simulink model "sampleModel1461"  (R2023a)
settings: Solver=VariableStepAuto  StartTime=0.0  StopTime=10.0  RelTol=1e-3
libraries: hdlsllib x6
settings Model: Creator=user1  LastModifiedBy=user1

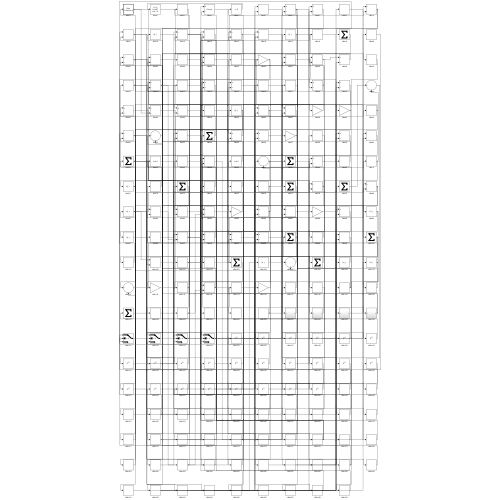
[thumbnail: Simulink's stored preview of the top-level diagram]
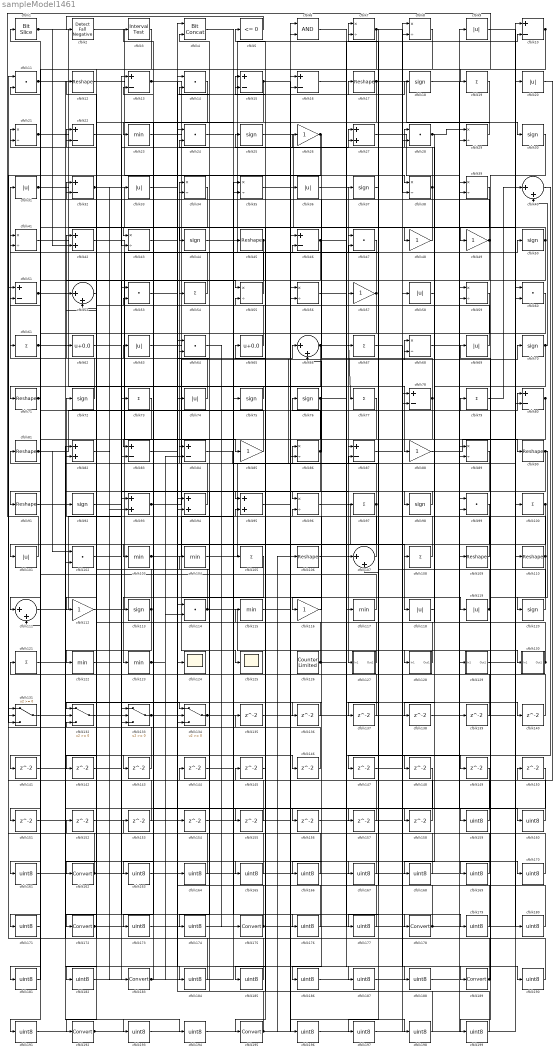
== system sampleModel1461 ==
  cfblk1 : hdlsllib/Logic and Bit Operations/Bit Slice  lidx=7  ridx=0
  cfblk{10,13,15..16,22,32,46,51,78,80,83..84,87} (13 alike) : Sum  Inputs=+-
  cfblk{19,54,61,67,73,77,79,97,100,105,108,121} (12 alike) : Sum  Inputs=+
  cfblk{9,20,31,33,36,58,63,69,74,101,118..119} (12 alike) : Abs  SaturateOnIntegerOverflow=off
  cfblk{11,14,24,28,47,53,60,64,99,102,114} (11 alike) : DotProduct  OutDataTypeStr=Inherit: Inherit via internal rule
  cfblk{23,103..104,115,117,122..123} (7 alike) : MinMax
  cfblk{12,17,45,71,81,90..91,106,109..110} (10 alike) : Reshape
  cfblk{40,52,66,107,111} (5 alike) : Sum  Inputs=|++
  cfblk{26,48..49,57,85,88,112,116} (8 alike) : Gain
  cfblk{18,25,30,37,44,50,70,72,75..76,92,98,113,120} (14 alike) : Signum
  cfblk124 : Scope
  cfblk125 : Scope
  cfblk126 : hdlsllib/Sources/Counter Limited  uplimit=7  tsamp=-1
  cfblk127 : Subsystem
      settings: LibrarySourceBlock=|
      | hdlsllib/Ports &
      | Subsystems/Subsystem
  cfblk128 : Subsystem
      settings: LibrarySourceBlock=|
      | hdlsllib/Ports &
      | Subsystems/Subsystem
  cfblk129 : Subsystem
      settings: LibrarySourceBlock=|
      | hdlsllib/Ports &
      | Subsystems/Subsystem
  cfblk130 : Subsystem
      settings: LibrarySourceBlock=|
      | hdlsllib/Ports &
      | Subsystems/Subsystem
  cfblk{131..134} (4 alike) : Switch  SaturateOnIntegerOverflow=off  InputSameDT=off
  cfblk{135..158} (24 alike) : Delay  SampleTime=1
  cfblk{159..161,163..171,173..174,176..177,179..182,184..188,190..191,193..194,196..199} (33 alike) : DataTypeConversion  OutDataTypeStr=uint8  SaturateOnIntegerOverflow=off  RndMeth=Floor
  cfblk{162,172,175,178,183,189,192,195} (8 alike) : DataTypeConversion  SaturateOnIntegerOverflow=off  RndMeth=Floor
  cfblk2 : hdlsllib/Logic and Bit Operations/Detect Fall Negative  vinit=0  OutDataTypeStr=boolean
  cfblk{7..8,21,29,34..35,38..39,41,43,55..56,59,68,86,89,96} (17 alike) : Product  Inputs=*/  RndMeth=Zero  SaturateOnIntegerOverflow=on
  cfblk{27,42,82,93..95} (6 alike) : Sum
  cfblk3 : hdlsllib/Logic and Bit Operations/Interval Test  IntervalClosedRight=on  uplimit=0.5  IntervalClosedLeft=on  lowlimit=-0.5  OutDataTypeStr=boolean
  cfblk4 : hdlsllib/Logic and Bit Operations/Bit Concat  numInputs=2
  cfblk5 : hdlsllib/Logic and Bit Operations/Compare To Zero  relop=<=  OutDataTypeStr=boolean
  cfblk6 : Logic  AllPortsSameDT=off  OutDataTypeStr=boolean
  cfblk62 : Bias  Bias=0.0  SaturateOnIntegerOverflow=off
  cfblk65 : Bias  Bias=0.0  SaturateOnIntegerOverflow=off
  wires:
  cfblk114/1 -> cfblk128/1(In1), cfblk62/1
  cfblk17/1 -> cfblk30/1, cfblk134/3
  cfblk45/1 -> cfblk151/1, cfblk163/1
  cfblk63/1 -> cfblk96/1
  cfblk120/1 -> cfblk86/1
  cfblk55/1 -> cfblk7/1
  cfblk42/1 -> cfblk85/1
  cfblk106/1 -> cfblk127/1(In1)
  cfblk84/1 -> cfblk68/1
  cfblk79/1 -> cfblk40/1
  cfblk110/1 -> cfblk72/1, cfblk169/1
  cfblk1/1 -> cfblk88/1, cfblk42/2
  cfblk23/1 -> cfblk125/1
  cfblk93/1 -> cfblk68/2, cfblk108/1
  cfblk107/1 -> cfblk5/1
  cfblk13/1 -> cfblk119/1, cfblk156/1, cfblk187/1
  cfblk50/1 -> cfblk107/1, cfblk49/1
  cfblk3/1 -> cfblk162/1
  cfblk39/1 -> cfblk195/1
  cfblk66/1 -> cfblk77/1, cfblk10/2, cfblk191/1
  cfblk14/1 -> cfblk172/1
  cfblk74/1 -> cfblk42/1
  cfblk104/1 -> cfblk20/1
  cfblk52/1 -> cfblk132/1
  cfblk12/1 -> cfblk38/1
  cfblk34/1 -> cfblk43/1
  cfblk25/1 -> cfblk48/1
  cfblk75/1 -> cfblk71/1
  cfblk113/1 -> cfblk32/2, cfblk142/1
  cfblk28/1 -> cfblk29/1, cfblk138/1
  cfblk116/1 -> cfblk96/2
  cfblk5/1 -> cfblk2/1
  cfblk65/1 -> cfblk21/1
  cfblk21/1 -> cfblk100/1, cfblk143/1
  cfblk94/1 -> cfblk12/1
  cfblk49/1 -> cfblk91/1, cfblk21/2
  cfblk38/1 -> cfblk25/1, cfblk171/1
  cfblk97/1 -> cfblk34/1, cfblk134/2
  cfblk32/1 -> cfblk124/1, cfblk93/2
  cfblk59/1 -> cfblk192/1
  cfblk130/1(Out1) -> cfblk27/1, cfblk28/1
  cfblk96/1 -> cfblk118/1
  cfblk37/1 -> cfblk107/2
  cfblk44/1 -> cfblk105/1
  cfblk72/1 -> cfblk31/1
  cfblk56/1 -> cfblk189/1
  cfblk82/1 -> cfblk183/1
  cfblk101/1 -> cfblk19/1
  cfblk133/1 -> cfblk74/1, cfblk66/1
  cfblk112/1 -> cfblk50/1
  cfblk80/1 -> cfblk182/1, cfblk185/1
  cfblk36/1 -> cfblk57/1
  cfblk51/1 -> cfblk146/1, cfblk176/1
  cfblk108/1 -> cfblk92/1
  cfblk105/1 -> cfblk123/1
  cfblk70/1 -> cfblk40/2, cfblk148/1
  cfblk86/1 -> cfblk66/2, cfblk76/1, cfblk133/3, cfblk174/1
  cfblk57/1 -> cfblk46/2, cfblk155/1
  cfblk77/1 -> cfblk87/1
  cfblk85/1 -> cfblk61/1
  cfblk22/1 -> cfblk43/2
  cfblk54/1 -> cfblk34/2
  cfblk15/1 -> cfblk103/1, cfblk157/1
  cfblk126/1 -> cfblk22/1, cfblk79/1
  cfblk91/1 -> cfblk97/1
  cfblk8/1 -> cfblk111/1
  cfblk64/1 -> cfblk175/1
  cfblk109/1 -> cfblk84/1
  cfblk41/1 -> cfblk94/2
  cfblk69/1 -> cfblk22/2
  cfblk111/1 -> cfblk33/1
  cfblk26/1 -> cfblk116/1, cfblk131/3
  cfblk123/1 -> cfblk63/1, cfblk84/2
  cfblk92/1 -> cfblk27/2
  cfblk117/1 -> cfblk41/1
  cfblk102/1 -> cfblk113/1
  cfblk78/1 -> cfblk112/1, cfblk32/1
  cfblk11/1 -> cfblk55/1, cfblk134/1
  cfblk33/1 -> cfblk15/1
  cfblk47/1 -> cfblk41/2
  cfblk88/1 -> cfblk90/1
  cfblk29/1 -> cfblk23/1
  cfblk68/1 -> cfblk29/2
  cfblk58/1 -> cfblk98/1
  cfblk98/1 -> cfblk95/1
  cfblk31/1 -> cfblk129/1(In1), cfblk188/1
  cfblk2/1 -> cfblk75/1
  cfblk119/1 -> cfblk26/1, cfblk87/2
  cfblk95/1 -> cfblk70/1
  cfblk48/1 -> cfblk44/1
  cfblk90/1 -> cfblk120/1, cfblk177/1
  cfblk43/1 -> cfblk114/1
  cfblk81/1 -> cfblk8/1, cfblk102/1, cfblk158/1
  cfblk7/1 -> cfblk38/2, cfblk47/1, cfblk52/2
  cfblk71/1 -> cfblk51/2, cfblk161/1
  cfblk100/1 -> cfblk102/2, cfblk141/1
  cfblk67/1 -> cfblk130/1(In1)
  cfblk128/1(Out1) -> cfblk95/2
  cfblk27/1 -> cfblk109/1
  cfblk103/1 -> cfblk35/2, cfblk17/1
  cfblk129/1(Out1) -> cfblk10/1
  cfblk46/1 -> cfblk133/2, cfblk140/1
  cfblk127/1(Out1) -> cfblk13/2
  cfblk60/1 -> cfblk101/1
  cfblk61/1 -> cfblk78/2, cfblk83/2, cfblk184/1
  cfblk132/1 -> cfblk80/1
  cfblk134/1 -> cfblk67/1, cfblk16/2, cfblk99/2
  cfblk19/1 -> cfblk122/1
  cfblk76/1 -> cfblk18/1, cfblk83/1
  cfblk10/1 -> cfblk28/2, cfblk137/1
  cfblk24/1 -> cfblk178/1
  cfblk135/1 -> cfblk60/2
  cfblk99/1 -> cfblk136/1
  cfblk136/1 -> cfblk132/2
  cfblk137/1 -> cfblk52/1
  cfblk138/1 -> cfblk80/2
  cfblk139/1 -> cfblk11/2
  cfblk140/1 -> cfblk15/2
  cfblk141/1 -> cfblk13/1
  cfblk142/1 -> cfblk133/1
  cfblk143/1 -> cfblk131/2
  cfblk144/1 -> cfblk35/1
  cfblk145/1 -> cfblk55/2
  cfblk146/1 -> cfblk132/3
  cfblk40/1 -> cfblk147/1
  cfblk147/1 -> cfblk78/1
  cfblk16/1 -> cfblk149/1
  cfblk20/1 -> cfblk150/1
  cfblk152/1 -> cfblk86/2
  cfblk153/1 -> cfblk131/1
  cfblk83/1 -> cfblk154/1
  cfblk154/1 -> cfblk46/1
  cfblk155/1 -> cfblk111/2
  cfblk156/1 -> cfblk8/2
  cfblk157/1 -> cfblk1/1
  cfblk158/1 -> cfblk7/2
  cfblk6/1 -> cfblk159/1
  cfblk159/1 -> cfblk65/1
  cfblk18/1 -> cfblk160/1
  cfblk160/1 -> cfblk6/1
  cfblk161/1 -> cfblk6/2
  cfblk162/1 -> cfblk152/1, cfblk9/1
  cfblk163/1 -> cfblk3/1
  cfblk53/1 -> cfblk164/1
  cfblk164/1 -> cfblk11/1
  cfblk122/1 -> cfblk165/1
  cfblk165/1 -> cfblk53/1
  cfblk148/1 -> cfblk166/1
  cfblk166/1 -> cfblk53/2
  cfblk4/1 -> cfblk167/1
  cfblk167/1 -> cfblk93/1
  cfblk118/1 -> cfblk168/1
  cfblk168/1 -> cfblk4/1
  cfblk169/1 -> cfblk4/2
  cfblk121/1 -> cfblk170/1
  cfblk170/1 -> cfblk135/1
  cfblk171/1 -> cfblk121/1
  cfblk172/1 -> cfblk37/1, cfblk60/1
  cfblk150/1 -> cfblk173/1
  cfblk173/1 -> cfblk14/1
  cfblk174/1 -> cfblk14/2
  cfblk175/1 -> cfblk145/1, cfblk144/1, cfblk117/1
  cfblk176/1 -> cfblk64/1
  cfblk177/1 -> cfblk64/2
  cfblk178/1 -> cfblk47/2, cfblk104/1, cfblk16/1
  cfblk62/1 -> cfblk179/1
  cfblk179/1 -> cfblk24/1
  cfblk9/1 -> cfblk180/1
  cfblk180/1 -> cfblk24/2
  cfblk73/1 -> cfblk181/1
  cfblk181/1 -> cfblk81/1
  cfblk182/1 -> cfblk73/1
  cfblk183/1 -> cfblk153/1, cfblk114/2, cfblk45/1
  cfblk184/1 -> cfblk82/1
  cfblk185/1 -> cfblk82/2
  cfblk89/1 -> cfblk186/1
  cfblk186/1 -> cfblk139/1
  cfblk187/1 -> cfblk89/1
  cfblk188/1 -> cfblk89/2
  cfblk189/1 -> cfblk51/1, cfblk69/1
  cfblk87/1 -> cfblk190/1
  cfblk190/1 -> cfblk56/1
  cfblk191/1 -> cfblk56/2
  cfblk192/1 -> cfblk36/1, cfblk110/1, cfblk99/1
  cfblk151/1 -> cfblk193/1
  cfblk193/1 -> cfblk59/1
  cfblk131/1 -> cfblk194/1
  cfblk194/1 -> cfblk59/2
  cfblk195/1 -> cfblk54/1, cfblk58/1, cfblk106/1
  cfblk35/1 -> cfblk196/1
  cfblk196/1 -> cfblk39/1
  cfblk149/1 -> cfblk197/1
  cfblk197/1 -> cfblk39/2
  cfblk115/1 -> cfblk198/1
  cfblk198/1 -> cfblk94/1
  cfblk30/1 -> cfblk199/1
  cfblk199/1 -> cfblk115/1

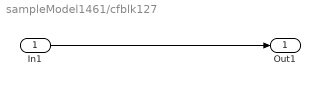
== system sampleModel1461/cfblk127 ==
  In1 : Inport
  Out1 : Outport
  wires:
  In1/1 -> Out1/1

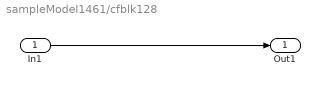
== system sampleModel1461/cfblk128 ==
  In1 : Inport
  Out1 : Outport
  wires:
  In1/1 -> Out1/1

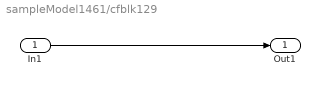
== system sampleModel1461/cfblk129 ==
  In1 : Inport
  Out1 : Outport
  wires:
  In1/1 -> Out1/1

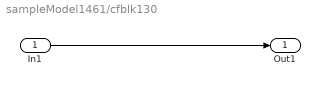
== system sampleModel1461/cfblk130 ==
  In1 : Inport
  Out1 : Outport
  wires:
  In1/1 -> Out1/1
